simulink subsystem "VoltageDriver_balrob"  (R2024b)
settings: Solver=VariableStepAuto  StartTime=0.0  StopTime=10.0  RelTol=1e-3
values from neighbouring files (symbols this model uses):
  Ts = 1e-2    (= 0.01)    [Plant_balrob_params.m]
undefined symbols (not defined in the file or in its folder): drv
settings Model: Creator=federico  LastModifiedBy=federico

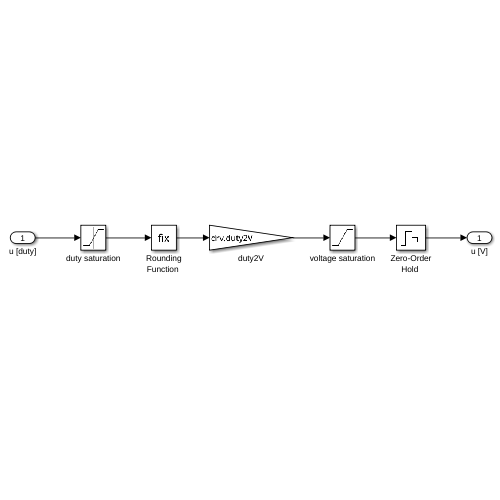
[thumbnail: Simulink's stored preview of the top-level diagram]
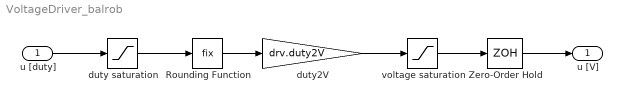
== system VoltageDriver_balrob ==
  u [duty] : Inport
  "Rounding Function " : Rounding  Operator=fix
  "Zero-Order Hold " : ZeroOrderHold  SampleTime=Ts
  duty saturation : Saturate  UpperLimit=drv.dutymax  LowerLimit=-drv.dutymax
  duty2V : Gain  Gain=drv.duty2V
  voltage saturation : Saturate  UpperLimit=drv.Vbus  LowerLimit=-drv.Vbus
  u [V] : Outport
  wires:
  u [duty]/1 -> duty saturation/1
  duty saturation/1 -> "Rounding Function "/1
  "Rounding Function "/1 -> duty2V/1
  duty2V/1 -> voltage saturation/1
  voltage saturation/1 -> "Zero-Order Hold "/1
  "Zero-Order Hold "/1 -> u [V]/1
